simulink model "FSKRaisedCosine"  (R2016a)
settings: Solver=VariableStepAuto  StartTime=0.0  StopTime=10.0  RelTol=1e-3
libraries: commdigbbndfm2 x2, commfilt2 x2, commchan3 x1, commsink2 x1, commrandsrc3 x1
settings Model: Creator=Omar  LastModifiedBy=Omar

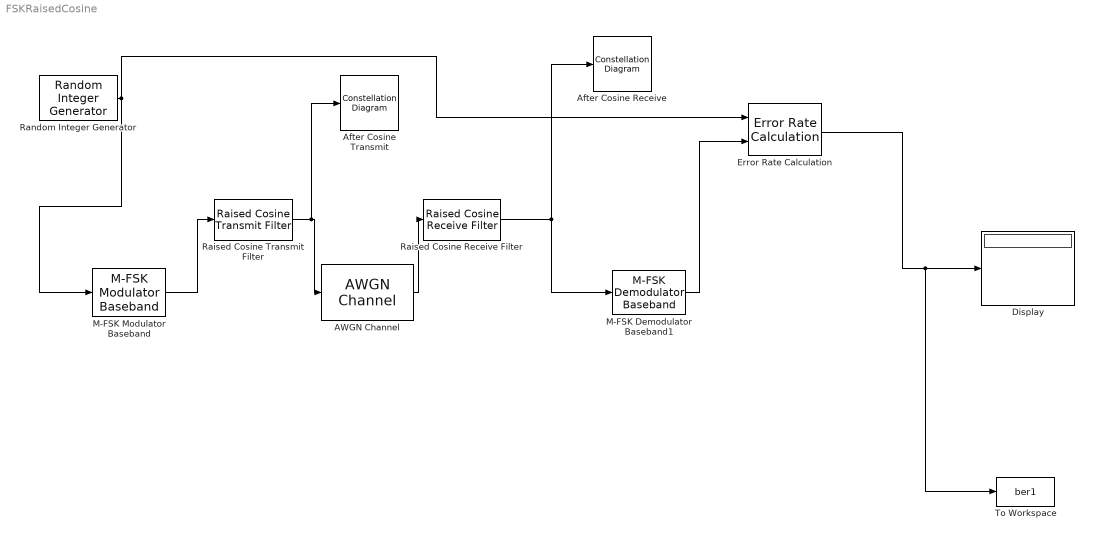
== system FSKRaisedCosine ==
  AWGN Channel : commchan3/AWGN Channel  InputProcessing=Columns as channels (frame based)  seed=67  noiseMode="Signal to noise ratio  (Eb/No)"  EbNodB=EbNo  EsNodB=10  SNRdB=10  bitsPerSym=1  Ps=1  Tsym=1  variance=1
  After Cosine Receive : ConstellationDiagram
  After Cosine Transmit : ConstellationDiagram
  Display : Display
  Error Rate Calculation : commsink2/Error Rate Calculation  N=8  st_delay=0  cp_mode=Entire frame  subframe=[]  PMode=Port  WsName=ErrorVec  RsMode2=off  stop=on  numErr=100  maxBits=1e6
  M-FSK Demodulator Baseband1 : commdigbbndfm2/M-FSK Demodulator Baseband  M=2  OutType=Integer  Dec=Gray  freqSep=6  numSamp=17  RateOptions=Enforce single-rate processing  outDataType=double
  M-FSK Modulator Baseband : commdigbbndfm2/M-FSK Modulator Baseband  M=2  InType=Integer  Enc=Gray  freqSep=6  phaseType=Continuous  numSamp=17  RateOptions=Enforce single-rate processing  outDataType=double
  Raised Cosine Receive Filter : commfilt2/Raised Cosine Receive Filter  filtType=Normal  R=0.2  filtSpan=10  N=8  downFactor=8  downOffset=0  filterGain=1  InputProcessing=Columns as channels (frame based)  RateOptions=Enforce single-rate processing  framing=Mute  checkCoeff=off  variableName=rcRxFilt  currentFiltSpan=10  D=5  inputOffset=0  sampMode=Mute  saveAsFlag=0  rateMode=Downsampling  checkGain=Normalized  launchFVT=on  roundingMode=Floor  overflowMode=off  coeffDataTypeStr=Inherit: Same word length as input  coeffMin=[]  coeffMax=[]  coeffLastDataTypeStr=Inherit: Same word length as input  accumDataTypeStr=Inherit: Same as product output  accumLastDataTypeStr=Inherit: Same as product output  outputDataTypeStr=Inherit: Same as accumulator  outputMin=[]  outputMax=[]  outputLastDataTypeStr=Inherit: Same as accumulator
  Raised Cosine Transmit Filter : commfilt2/Raised Cosine Transmit Filter  filtType=Normal  R=0.2  filtSpan=8  N=8  filterGain=1  InputProcessing=Columns as channels (frame based)  RateOptions=Enforce single-rate processing  framing=Mute  checkCoeff=off  variableName=rcTxFilt  checkGain=Normalized  sampMode=Mute  saveAsFlag=0  currentFiltSpan=8  D=(8)/2  launchFVT=on  roundingMode=Floor  overflowMode=off  coeffDataTypeStr=Inherit: Same word length as input  coeffMin=[]  coeffMax=[]  coeffLastDataTypeStr=Inherit: Same word length as input  outputDataTypeStr=Inherit: Same as accumulator  outputMin=[]  outputMax=[]  outputLastDataTypeStr=Inherit: Same as accumulator
  Random Integer Generator : commrandsrc3/Random Integer Generator  SetSize=2  SeedSource=Parameter  Seed=15  SampleTime=1  SamplesPerFrame=1  OutputDataType=double  SimulateUsing=Interpreted execution
  To Workspace : ToWorkspace  VariableName=ber1  SampleTime=-1
      settings: MaxDataPoints=2  Save2DSignal=2-D array (concatenate along first dimension)
  wires:
  Random Integer Generator/1 -> M-FSK Modulator Baseband/1, Error Rate Calculation/1
  M-FSK Demodulator Baseband1/1 -> Error Rate Calculation/2
  M-FSK Modulator Baseband/1 -> Raised Cosine Transmit Filter/1
  Raised Cosine Transmit Filter/1 -> After Cosine Transmit/1, AWGN Channel/1
  AWGN Channel/1 -> Raised Cosine Receive Filter/1
  Raised Cosine Receive Filter/1 -> M-FSK Demodulator Baseband1/1, After Cosine Receive/1
  Error Rate Calculation/1 -> To Workspace/1, Display/1
